simulink model "mobrob_mdl"  (R2022a)
settings: Solver=VariableStepAuto  StartTime=0.0  StopTime=9  RelTol=1e-3
values from neighbouring files (symbols this model uses):
  ell = 0.1    [mobrob_init.m]
  J_B = 0.01    [mobrob_init.m]
  K_kont = 1e6    (= 1000000)    [mobrob_init.m]
  m = 0.1    [mobrob_init.m]
  mg = m*g    (= 1)    [mobrob_init.m]
  Rr = 20e-3    (= 0.02)    [mobrob_init.m]
settings Model: Creator=bin3  LastModifiedBy=bin3

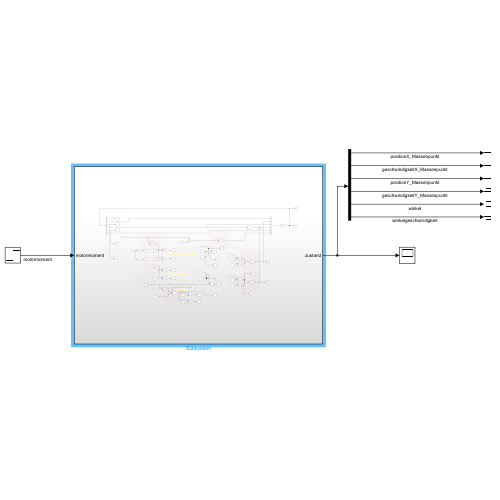
[thumbnail: Simulink's stored preview of the top-level diagram]
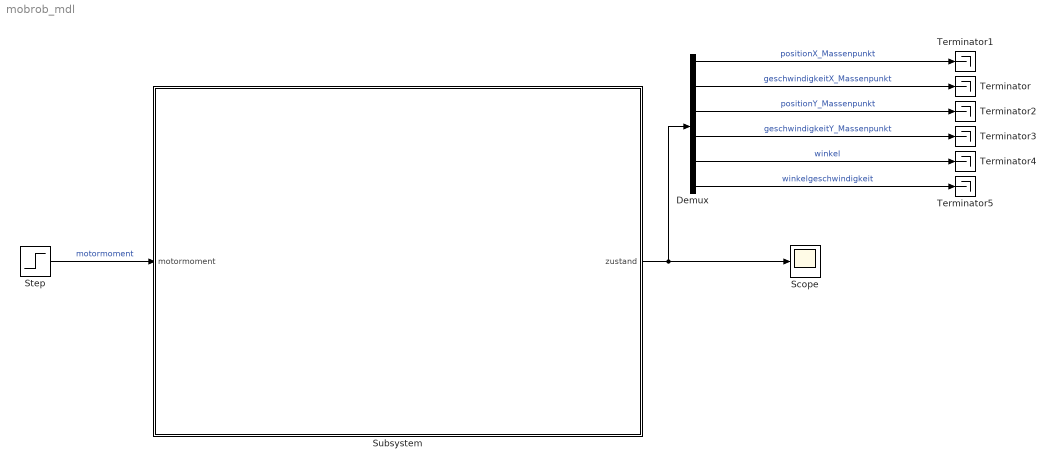
== system mobrob_mdl ==
  Demux : Demux  Outputs=6
  Scope : Scope
  Step : Step  SampleTime=0
  Subsystem : Subsystem
  Terminator{,1..5} (6 alike) : Terminator
  wires:
  Step/1 -> Subsystem/1(motormoment)  "motormoment"
  Subsystem/1(zustand) -> Scope/1, Demux/1
  Demux/2 -> Terminator/1  "geschwindigkeitX_Massenpunkt"
  Demux/1 -> Terminator1/1  "positionX_Massenpunkt"
  Demux/3 -> Terminator2/1  "positionY_Massenpunkt"
  Demux/4 -> Terminator3/1  "geschwindigkeitY_Massenpunkt"
  Demux/5 -> Terminator4/1  "winkel"
  Demux/6 -> Terminator5/1  "winkelgeschwindigkeit"

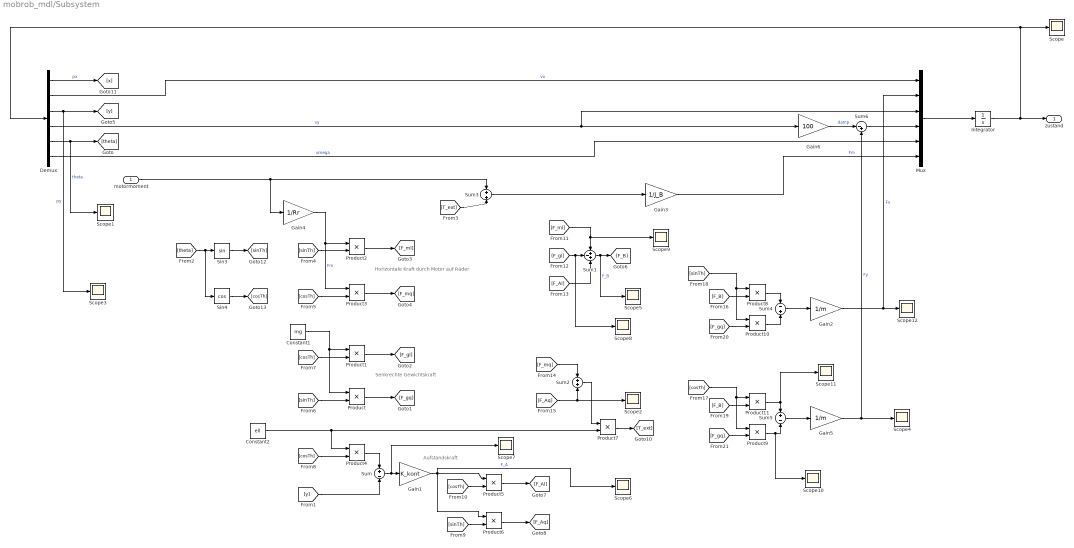
== system mobrob_mdl/Subsystem ==
  note: Horizontale Kraft durch Motor auf Räder
  note: Senkrechte Gewichtskraft
  note: Aufstandskraft
  motormoment : Inport
  Constant1 : Constant  Value=mg
  Constant2 : Constant  Value=ell
  Demux : Demux  Outputs=6
  Gain1 : Gain  Gain=K_kont
  Gain2 : Gain  Gain=1/m
  Gain3 : Gain  Gain=1/J_B
  Gain4 : Gain  Gain=1/Rr
  Gain5 : Gain  Gain=1/m
  Gain6 : Gain  Gain=100
  Integrator : Integrator  InitialCondition=[0 0 0.1 0 0.0000 0]
  Mux : Mux  Inputs=6
  Product{,1..11} (12 alike) : Product
  Scope{,1..12} (13 alike) : Scope
  Sin3 : Trigonometry
  Sin4 : Trigonometry  Operator=cos
  Sum : Sum  Inputs=+|-
  Sum1 : Sum  Inputs=+-+
  Sum2 : Sum  Inputs=+|+
  Sum3 : Sum  Inputs=+|+
  Sum4 : Sum  Inputs=-|+
  Sum5 : Sum  Inputs=+|-
  Sum6 : Sum  Inputs=|-+
  zustand : Outport
  wires:
  Gain2/1 -> Scope12/1, Mux/2  "Fx"
  [y] -> Sum/2
  Sin4/1 -> [cosTh]
  Product/1 -> [F_gq]
  Gain1/1 -> Scope6/1, Product6/1, Product5/1  "F_A"
  [F_ml] -> Scope9/1, Sum1/1
  Constant1/1 -> Product1/1, Product/1
  Demux/2 -> Mux/1  "vx"
  Sum/1 -> Scope7/1, Gain1/1
  Product4/1 -> Sum/1
  Mux/1 -> Integrator/1
  [theta] -> Sin3/1, Sin4/1
  Constant2/1 -> Product7/2, Product4/1
  [F_Al] -> Sum1/3
  [T_ext] -> Sum3/2
  Product10/1 -> Sum4/2
  Product9/1 -> Scope10/1, Sum5/2
  Integrator/1 -> zustand/1, Scope/1, Demux/1
  Demux/4 -> Gain6/1, Mux/3  "vy"
  Product2/1 -> [F_ml]
  [sinTh] -> Product6/2
  Product6/1 -> [F_Aq]
  Demux/6 -> Mux/5  "omega"
  [F_B] -> Product8/2
  Demux/5 -> Scope1/1, [theta]  "theta"
  [F_gq] -> Product10/2
  [sinTh] -> Product10/1, Product8/1
  Sum6/1 -> Mux/4
  Product5/1 -> [F_Al]
  Gain4/1 -> Product3/1, Product2/1  "Fm"
  Sum5/1 -> Gain5/1
  [cosTh] -> Product1/2
  Product1/1 -> [F_gl]
  Gain3/1 -> Mux/6  "Fm"
  Gain5/1 -> Scope4/1, Sum6/2  "Fy"
  [F_gq] -> Product9/2
  Product3/1 -> [F_mq]
  [sinTh] -> Product2/2
  [sinTh] -> Product/2
  Sum4/1 -> Gain2/1
  Sum3/1 -> Gain3/1
  [F_gl] -> Scope8/1, Sum1/2
  Demux/1 -> [x]  "px"
  Product7/1 -> [T_ext]
  [cosTh] -> Product9/1, Product11/1
  Demux/3 -> Scope3/1, [y]  "py"
  Sum1/1 -> Scope5/1, [F_B]  "F_B"
  Sum2/1 -> Product7/1
  [cosTh] -> Product4/2
  [F_mq] -> Sum2/1
  Sin3/1 -> [sinTh]
  [cosTh] -> Product5/2
  Gain6/1 -> Sum6/1  "damp"
  Product11/1 -> Scope11/1, Sum5/1
  Product8/1 -> Sum4/1
  [F_Aq] -> Scope2/1, Sum2/2
  [cosTh] -> Product3/2
  motormoment/1 -> Gain4/1, Sum3/1
  [F_B] -> Product11/2
